simulink model "sampleModel4"  (R2022a)
settings: Solver=VariableStepAuto  StartTime=0.0  StopTime=10.0  RelTol=1e-3
undefined symbols (not defined in the file): DiscIntNeverNeededParam, magnitude, Newton, Raphson
libraries: simulink x90, slpidlib x34
(part 1 of 4)
settings Model: Creator=TSMC  LastModifiedBy=TSMC

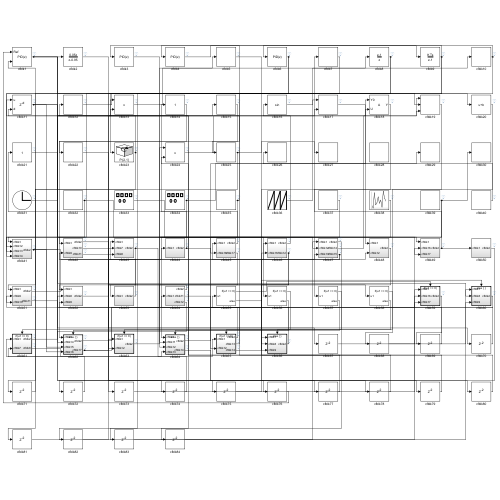
[thumbnail: Simulink's stored preview of the top-level diagram]
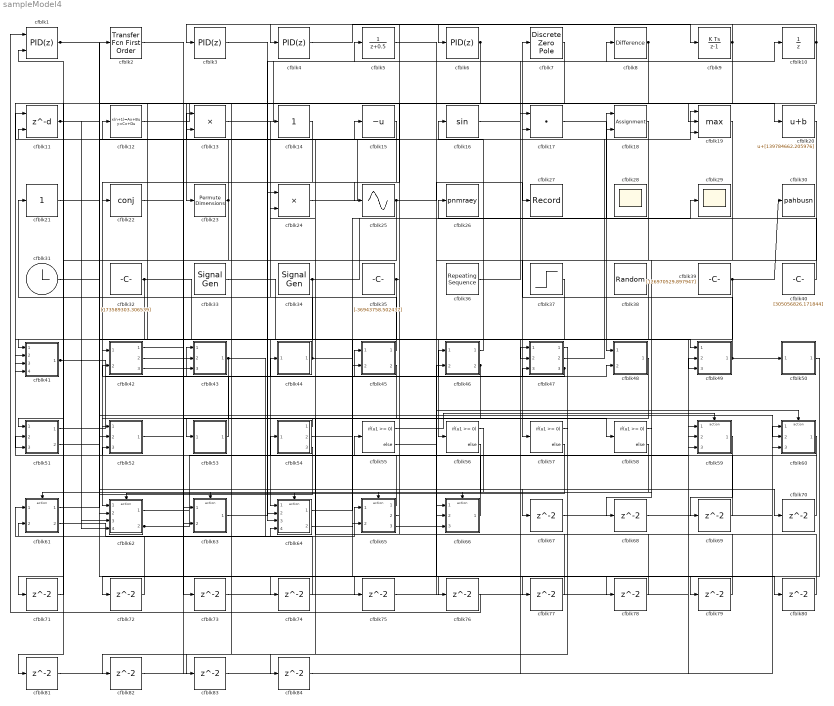
== system sampleModel4 ==
  cfblk1 : slpidlib/PID Controller (2DOF)  Controller=PID  Form=Parallel  TimeDomain=Discrete-time  UseExternalTs=off  SampleTime=1  IntegratorMethod=Forward Euler  FilterMethod=Forward Euler  ControllerParametersSource=internal  P=1  I=1  UseKiTs=off  D=0  N=100  UseFilter=on  b=1  c=1  TunerSelectOption=Transfer Function Based (PID Tuner App)  InitialConditionSource=internal  InitialConditionForIntegrator=0  InitialConditionForFilter=0  DifferentiatorICPrevScaledInput=0  ExternalReset=none  TrackingMode=off  Kt=1  LimitOutput=off  SatLimitsSource=internal  UpperSaturationLimit=inf  LowerSaturationLimit=-inf  LinearizeAsGain=off  AntiWindupMode=none  Kb=1  POutMin=[]  POutMax=[]  IOutMin=[]  IOutMax=[]  DOutMin=[]  DOutMax=[]  NOutMin=[]  NOutMax=[]  bOutMin=[]  bOutMax=[]  cOutMin=[]  cOutMax=[]  SumOutMin=[]  SumOutMax=[]  SaturationOutMin=[]  SaturationOutMax=[]  PParamMin=[]  PParamMax=[]  IParamMin=[]  IParamMax=[]  DParamMin=[]  DParamMax=[]  NParamMin=[]  NParamMax=[]  bParamMin=[]  bParamMax=[]  cParamMin=[]  cParamMax=[]  KbParamMin=[]  KbParamMax=[]  KtParamMin=[]  KtParamMax=[]  KbOutMin=[]  KbOutMax=[]  KtOutMin=[]  KtOutMax=[]  IntegratorOutMin=[]  IntegratorOutMax=[]  FilterOutMin=[]  FilterOutMax=[]  SumI1OutMin=[]  SumI1OutMax=[]  SumI2OutMin=[]  SumI2OutMax=[]  SumI3OutMin=[]  SumI3OutMax=[]  SumI4OutMin=[]  SumI4OutMax=[]  SumDOutMin=[]  SumDOutMax=[]  Sum1OutMin=[]  Sum1OutMax=[]  Sum2OutMin=[]  Sum2OutMax=[]  Sum3OutMin=[]  Sum3OutMax=[]  DifferentiatorOutMin=[]  DifferentiatorOutMax=[]  FilterDiffOutCoefMin=[]  FilterDiffOutCoefMax=[]  ReciprocalOutMin=[]  ReciprocalOutMax=[]  SumDenOutMin=[]  SumDenOutMax=[]  SumNumOutMin=[]  SumNumOutMax=[]  DivideOutMin=[]  DivideOutMax=[]  UdiffTsProdOutMin=[]  UdiffTsProdOutMax=[]  NTsProdOutMin=[]  NTsProdOutMax=[]  UintegralTsProdOutMin=[]  UintegralTsProdOutMax=[]  UngainTsProdOutMin=[]  UngainTsProdOutMax=[]  IntegratorContinuousStateAttributes=''  IntegratorStateMustResolveToSignalObject=off  IntegratorRTWStateStorageClass=Auto  FilterContinuousStateAttributes=''  FilterStateMustResolveToSignalObject=off  FilterRTWStateStorageClass=Auto  ParallelPVariant=InternalParameters  IdealPVariant=Disabled  IVariant=InternalParameters  DVariant=InternalParameters  bVariant=InternalParameters  cVariant=InternalParameters  IntegratorVariant=Discrete  SatVariant=Disabled  AWVariant=Passthrough  PCopyVariant=Disabled  TRVariant=Disabled  FdbkBlocksVariant=Forward  IdealPFdbkVariant=Disabled  SatFdbkVariant=Disabled  DerivativeFilterVariant=ForwardEulerFilter  NVariant=InternalParameters  NCopyVariant=Disabled  FilterICVariant=InternalICsFilter  IntegratorICVariant=InternalICs  ExternalResetVariant=Disabled  TRSumVariant=Passthrough  SumFdbkVariant=Disabled  SumVariant=Sum_PID  TsampFilterVariant=InternalTs  TsampNgainVariant=Passthrough  TsampIntegralVariant=Passthrough  ExternalSaturationOutDataTypeStr=Inherit: Same as second input
      settings: SourceProductBaseCode=SL
  cfblk10 : UnitDelay  HasFrameUpgradeWarning=on
  cfblk11 : Delay  DelayLengthSource=Input port  SampleTime=1
      settings: InputPortMap=u0,p1
  cfblk12 : DiscreteStateSpace
  cfblk13 : Product  Inputs=**
  cfblk14 : simulink/Math Operations/Slider Gain  gain=1  low=0  high=2
  cfblk15 : UnaryMinus
  cfblk16 : Trigonometry
  cfblk17 : DotProduct  OutDataTypeStr=Inherit: Inherit via internal rule
  cfblk18 : Assignment  DiagnosticForDimensions=Warning  IndexOptions=Index vector (dialog)  Indices=1  OutputSizes=1
  cfblk19 : MinMax  Function=max  Inputs=3
  cfblk2 : simulink/Discrete/Transfer Fcn First Order  PoleZ=0.95  ICPrevOutput=0.0  DoSatur=off
  cfblk20 : Bias  Bias=[139784662.205976]  SaturateOnIntegerOverflow=off
  cfblk21 : simulink/Math Operations/Slider Gain  gain=1  low=0  high=2
  cfblk22 : Math  Operator=conj
  cfblk23 : PermuteDimensions
  cfblk24 : Product  Inputs=**
  cfblk25 : Sin  TimeSource=Use external signal  SampleTime=0
  cfblk26 : ToWorkspace  VariableName=pnmraey  SaveFormat=Timeseries  SampleTime=-1
  cfblk27 : Record  FileSettingsInternal="{\"entries\":[{\"content\":{\"excelSettings\":{\"content\":{},\"type\":\"Streamout.ExcelSettings\"}},\"type\":\"Streamout.FileSettingStorage\",\"uuid\":\"17087479-7456-49d2-b213-c1ed72e334c6\"}],\"packageUris\":[\"http://schema.mathworks.com/mf0/streamout_blocks/R2020a\"],\"version\":\"1.0\"}"  SignalsInternal="{\"entries\":[{\"content\":{\"signals\":[{\"content\":{\"blockPath\":[\"sampleModel4/cfblk27\"],\"channel\":[],\"dimensions\":[1],\"domain\":\"sampleModel4/cfblk27\",\"lineColor\":\"#fe330a\",\"plots\":[1],\"port\":1,\"sid\":[\"\"],\"signalID\":1694,\"signalName\":\"cfblk25\"},\"type\":\"RecordBlkView.Signal\",\"uuid\":\"3c895155-84a9-4b62-997f-1b293a1a0065\"}]},\"type\":\"RecordBlkView.InputSignals\",\"uuid\":\"3ad74f41-9a96-40a9-a38d-74122b75e475\"}],\"packageUris\":[\"http://schema.mathworks.com/mf0/streamout_blocks/R2020a\"],\"version\":\"1.0\"}"  VisualizationBindings="{\"sparklinesplugin\":{\"info\":[{\"bindingParametersList\":[],\"subplotID\":1}]}}"
  cfblk28 : Scope
      settings: Floating=on
  cfblk29 : Scope
  cfblk3 : slpidlib/PID Controller  Controller=PID  Form=Parallel  TimeDomain=Discrete-time  UseExternalTs=off  SampleTime=1  IntegratorMethod=Forward Euler  FilterMethod=Forward Euler  ControllerParametersSource=internal  P=1  I=1  UseKiTs=off  D=0  N=100  UseFilter=on  TunerSelectOption=Transfer Function Based (PID Tuner App)  InitialConditionSource=internal  InitialConditionForIntegrator=0  InitialConditionForFilter=0  DifferentiatorICPrevScaledInput=0  ExternalReset=none  TrackingMode=off  Kt=1  LimitOutput=off  SatLimitsSource=internal  UpperSaturationLimit=inf  LowerSaturationLimit=-inf  LinearizeAsGain=off  AntiWindupMode=none  Kb=1  POutMin=[]  POutMax=[]  IOutMin=[]  IOutMax=[]  DOutMin=[]  DOutMax=[]  NOutMin=[]  NOutMax=[]  SumOutMin=[]  SumOutMax=[]  SaturationOutMin=[]  SaturationOutMax=[]  PParamMin=[]  PParamMax=[]  IParamMin=[]  IParamMax=[]  DParamMin=[]  DParamMax=[]  NParamMin=[]  NParamMax=[]  KbParamMin=[]  KbParamMax=[]  KtParamMin=[]  KtParamMax=[]  KbOutMin=[]  KbOutMax=[]  KtOutMin=[]  KtOutMax=[]  IntegratorOutMin=[]  IntegratorOutMax=[]  FilterOutMin=[]  FilterOutMax=[]  SumI1OutMin=[]  SumI1OutMax=[]  SumI2OutMin=[]  SumI2OutMax=[]  SumI3OutMin=[]  SumI3OutMax=[]  SumI4OutMin=[]  SumI4OutMax=[]  SumDOutMin=[]  SumDOutMax=[]  DifferentiatorOutMin=[]  DifferentiatorOutMax=[]  FilterDiffOutCoefMin=[]  FilterDiffOutCoefMax=[]  ReciprocalOutMin=[]  ReciprocalOutMax=[]  SumDenOutMin=[]  SumDenOutMax=[]  SumNumOutMin=[]  SumNumOutMax=[]  DivideOutMin=[]  DivideOutMax=[]  UdiffTsProdOutMin=[]  UdiffTsProdOutMax=[]  NTsProdOutMin=[]  NTsProdOutMax=[]  UintegralTsProdOutMin=[]  UintegralTsProdOutMax=[]  UngainTsProdOutMin=[]  UngainTsProdOutMax=[]  IntegratorContinuousStateAttributes=''  IntegratorStateMustResolveToSignalObject=off  IntegratorRTWStateStorageClass=Auto  FilterContinuousStateAttributes=''  FilterStateMustResolveToSignalObject=off  FilterRTWStateStorageClass=Auto  ParallelPVariant=InternalParameters  IdealPVariant=Disabled  IVariant=InternalParameters  DVariant=InternalParameters  IntegratorVariant=Discrete  SatVariant=Disabled  AWVariant=Passthrough  PCopyVariant=Disabled  TRVariant=Disabled  FdbkBlocksVariant=Forward  IdealPFdbkVariant=Disabled  SatFdbkVariant=Disabled  DerivativeFilterVariant=ForwardEulerFilter  NVariant=InternalParameters  NCopyVariant=Disabled  FilterICVariant=InternalICsFilter  IntegratorICVariant=InternalICs  ExternalResetVariant=Disabled  TRSumVariant=Passthrough  SumFdbkVariant=Disabled  SumVariant=Sum_PID  TsampFilterVariant=InternalTs  TsampNgainVariant=Passthrough  TsampIntegralVariant=Passthrough  ExternalSaturationOutDataTypeStr=Inherit: Same as second input  aMode=0
  cfblk30 : ToWorkspace  VariableName=pahbusn  SaveFormat=Timeseries  SampleTime=-1
  cfblk31 : Clock
  cfblk32 : Constant  Value=[173589303.306539]  SampleTime=1
  cfblk33 : SignalGenerator  WaveForm=square  Amplitude=[-172169984.241983]
  cfblk34 : SignalGenerator  WaveForm=square  Amplitude=[319821277.257385]
  cfblk35 : Constant  Value=[-36943758.502437]  SampleTime=1
  cfblk36 : simulink/Sources/Repeating Sequence  rep_seq_t=[0 2]  rep_seq_y=[462391417.037504, 938938528.441266]
  cfblk37 : Step  Time=[19.000000]  Before=[-522799793.188864]  After=[-514590504.970175]  SampleTime=0
  cfblk38 : UniformRandomNumber  Minimum=[-9810606010.362951]  Maximum=[9826531795.280075]  Seed=[80261952.000000]  SampleTime=0.1
  cfblk39 : Constant  Value=[126970529.897947]  SampleTime=1
  cfblk4 : slpidlib/PID Controller  Controller=PID  Form=Parallel  TimeDomain=Discrete-time  UseExternalTs=off  SampleTime=1  IntegratorMethod=Forward Euler  FilterMethod=Forward Euler  ControllerParametersSource=internal  P=1  I=1  UseKiTs=off  D=0  N=100  UseFilter=on  TunerSelectOption=Transfer Function Based (PID Tuner App)  InitialConditionSource=internal  InitialConditionForIntegrator=0  InitialConditionForFilter=0  DifferentiatorICPrevScaledInput=0  ExternalReset=none  TrackingMode=off  Kt=1  LimitOutput=off  SatLimitsSource=internal  UpperSaturationLimit=inf  LowerSaturationLimit=-inf  LinearizeAsGain=off  AntiWindupMode=none  Kb=1  POutMin=[]  POutMax=[]  IOutMin=[]  IOutMax=[]  DOutMin=[]  DOutMax=[]  NOutMin=[]  NOutMax=[]  SumOutMin=[]  SumOutMax=[]  SaturationOutMin=[]  SaturationOutMax=[]  PParamMin=[]  PParamMax=[]  IParamMin=[]  IParamMax=[]  DParamMin=[]  DParamMax=[]  NParamMin=[]  NParamMax=[]  KbParamMin=[]  KbParamMax=[]  KtParamMin=[]  KtParamMax=[]  KbOutMin=[]  KbOutMax=[]  KtOutMin=[]  KtOutMax=[]  IntegratorOutMin=[]  IntegratorOutMax=[]  FilterOutMin=[]  FilterOutMax=[]  SumI1OutMin=[]  SumI1OutMax=[]  SumI2OutMin=[]  SumI2OutMax=[]  SumI3OutMin=[]  SumI3OutMax=[]  SumI4OutMin=[]  SumI4OutMax=[]  SumDOutMin=[]  SumDOutMax=[]  DifferentiatorOutMin=[]  DifferentiatorOutMax=[]  FilterDiffOutCoefMin=[]  FilterDiffOutCoefMax=[]  ReciprocalOutMin=[]  ReciprocalOutMax=[]  SumDenOutMin=[]  SumDenOutMax=[]  SumNumOutMin=[]  SumNumOutMax=[]  DivideOutMin=[]  DivideOutMax=[]  UdiffTsProdOutMin=[]  UdiffTsProdOutMax=[]  NTsProdOutMin=[]  NTsProdOutMax=[]  UintegralTsProdOutMin=[]  UintegralTsProdOutMax=[]  UngainTsProdOutMin=[]  UngainTsProdOutMax=[]  IntegratorContinuousStateAttributes=''  IntegratorStateMustResolveToSignalObject=off  IntegratorRTWStateStorageClass=Auto  FilterContinuousStateAttributes=''  FilterStateMustResolveToSignalObject=off  FilterRTWStateStorageClass=Auto  ParallelPVariant=InternalParameters  IdealPVariant=Disabled  IVariant=InternalParameters  DVariant=InternalParameters  IntegratorVariant=Discrete  SatVariant=Disabled  AWVariant=Passthrough  PCopyVariant=Disabled  TRVariant=Disabled  FdbkBlocksVariant=Forward  IdealPFdbkVariant=Disabled  SatFdbkVariant=Disabled  DerivativeFilterVariant=ForwardEulerFilter  NVariant=InternalParameters  NCopyVariant=Disabled  FilterICVariant=InternalICsFilter  IntegratorICVariant=InternalICs  ExternalResetVariant=Disabled  TRSumVariant=Passthrough  SumFdbkVariant=Disabled  SumVariant=Sum_PID  TsampFilterVariant=InternalTs  TsampNgainVariant=Passthrough  TsampIntegralVariant=Passthrough  ExternalSaturationOutDataTypeStr=Inherit: Same as second input  aMode=0
  cfblk40 : Constant  Value=[305056826.171844]  SampleTime=1
  cfblk41 : Subsystem
  cfblk42 : Subsystem
  cfblk43 : Subsystem
  cfblk44 : Subsystem
  cfblk45 : Subsystem
  cfblk46 : Subsystem
  cfblk47 : Subsystem
  cfblk48 : Subsystem
  cfblk49 : Subsystem
  cfblk5 : DiscreteTransferFcn  SampleTime=1
  cfblk50 : Subsystem
  cfblk51 : Subsystem
  cfblk52 : Subsystem
  cfblk53 : Subsystem
  cfblk54 : Subsystem
  cfblk{55..58} (4 alike) : If  IfExpression=u1 >= 0  SampleTime=1
  cfblk59 : Subsystem  TreatAsAtomicUnit=on
  cfblk6 : slpidlib/PID Controller  Controller=PID  Form=Parallel  TimeDomain=Discrete-time  UseExternalTs=off  SampleTime=1  IntegratorMethod=Forward Euler  FilterMethod=Forward Euler  ControllerParametersSource=internal  P=1  I=1  UseKiTs=off  D=0  N=100  UseFilter=on  TunerSelectOption=Transfer Function Based (PID Tuner App)  InitialConditionSource=internal  InitialConditionForIntegrator=0  InitialConditionForFilter=0  DifferentiatorICPrevScaledInput=0  ExternalReset=none  TrackingMode=off  Kt=1  LimitOutput=off  SatLimitsSource=internal  UpperSaturationLimit=inf  LowerSaturationLimit=-inf  LinearizeAsGain=off  AntiWindupMode=none  Kb=1  POutMin=[]  POutMax=[]  IOutMin=[]  IOutMax=[]  DOutMin=[]  DOutMax=[]  NOutMin=[]  NOutMax=[]  SumOutMin=[]  SumOutMax=[]  SaturationOutMin=[]  SaturationOutMax=[]  PParamMin=[]  PParamMax=[]  IParamMin=[]  IParamMax=[]  DParamMin=[]  DParamMax=[]  NParamMin=[]  NParamMax=[]  KbParamMin=[]  KbParamMax=[]  KtParamMin=[]  KtParamMax=[]  KbOutMin=[]  KbOutMax=[]  KtOutMin=[]  KtOutMax=[]  IntegratorOutMin=[]  IntegratorOutMax=[]  FilterOutMin=[]  FilterOutMax=[]  SumI1OutMin=[]  SumI1OutMax=[]  SumI2OutMin=[]  SumI2OutMax=[]  SumI3OutMin=[]  SumI3OutMax=[]  SumI4OutMin=[]  SumI4OutMax=[]  SumDOutMin=[]  SumDOutMax=[]  DifferentiatorOutMin=[]  DifferentiatorOutMax=[]  FilterDiffOutCoefMin=[]  FilterDiffOutCoefMax=[]  ReciprocalOutMin=[]  ReciprocalOutMax=[]  SumDenOutMin=[]  SumDenOutMax=[]  SumNumOutMin=[]  SumNumOutMax=[]  DivideOutMin=[]  DivideOutMax=[]  UdiffTsProdOutMin=[]  UdiffTsProdOutMax=[]  NTsProdOutMin=[]  NTsProdOutMax=[]  UintegralTsProdOutMin=[]  UintegralTsProdOutMax=[]  UngainTsProdOutMin=[]  UngainTsProdOutMax=[]  IntegratorContinuousStateAttributes=''  IntegratorStateMustResolveToSignalObject=off  IntegratorRTWStateStorageClass=Auto  FilterContinuousStateAttributes=''  FilterStateMustResolveToSignalObject=off  FilterRTWStateStorageClass=Auto  ParallelPVariant=InternalParameters  IdealPVariant=Disabled  IVariant=InternalParameters  DVariant=InternalParameters  IntegratorVariant=Discrete  SatVariant=Disabled  AWVariant=Passthrough  PCopyVariant=Disabled  TRVariant=Disabled  FdbkBlocksVariant=Forward  IdealPFdbkVariant=Disabled  SatFdbkVariant=Disabled  DerivativeFilterVariant=ForwardEulerFilter  NVariant=InternalParameters  NCopyVariant=Disabled  FilterICVariant=InternalICsFilter  IntegratorICVariant=InternalICs  ExternalResetVariant=Disabled  TRSumVariant=Passthrough  SumFdbkVariant=Disabled  SumVariant=Sum_PID  TsampFilterVariant=InternalTs  TsampNgainVariant=Passthrough  TsampIntegralVariant=Passthrough  ExternalSaturationOutDataTypeStr=Inherit: Same as second input  aMode=0
  cfblk60 : Subsystem  TreatAsAtomicUnit=on
  cfblk61 : Subsystem  TreatAsAtomicUnit=on
  cfblk62 : Subsystem  TreatAsAtomicUnit=on
  cfblk63 : Subsystem  TreatAsAtomicUnit=on
  cfblk64 : Subsystem  TreatAsAtomicUnit=on
  cfblk65 : Subsystem  TreatAsAtomicUnit=on
  cfblk66 : Subsystem  TreatAsAtomicUnit=on
  cfblk{67..84} (18 alike) : Delay  SampleTime=1
  cfblk7 : DiscreteZeroPole  Poles=[0 0.5]  Gain=1
  cfblk8 : simulink/Discrete/Difference  ICPrevInput=0.0  OutMin=[]  OutMax=[]  OutDataTypeStr=Inherit: Inherit via back propagation  OutDataType=fixdt(1, 16)  OutScaling=2^-10  DoSatur=off
  cfblk9 : DiscreteIntegrator  ICPrevOutput=DiscIntNeverNeededParam  ICPrevScaledInput=DiscIntNeverNeededParam
  wires:
  cfblk34/1 -> cfblk64/1(cfblk1), cfblk18/1
  cfblk66/1(cfblk2) -> cfblk12/1
  cfblk43/1(cfblk2) -> cfblk65/1(cfblk1), cfblk63/2(cfblk12)
  cfblk13/1 -> cfblk5/1
  cfblk35/1 -> cfblk3/1, cfblk43/2(cfblk7)
  cfblk38/1 -> cfblk64/2(cfblk11)
  cfblk40/1 -> cfblk26/1
  cfblk45/1(cfblk2) -> cfblk14/1
  cfblk44/1(cfblk2) -> cfblk21/1, cfblk79/1
  cfblk8/1 -> cfblk23/1, cfblk81/1
  cfblk49/1(cfblk2) -> cfblk7/1, cfblk50/1(cfblk1)
  cfblk4/1 -> cfblk9/1
  cfblk14/1 -> cfblk62/1(cfblk1)
  cfblk32/1 -> cfblk56/1, cfblk41/4(cfblk14)
  cfblk18/1 -> cfblk57/1
  cfblk53/1(cfblk2) -> cfblk43/1(cfblk1)
  cfblk60/1(cfblk2) -> cfblk54/1(cfblk1)
  cfblk51/1(cfblk2) -> cfblk44/1(cfblk1)
  cfblk48/1(cfblk2) -> cfblk64/3(cfblk12)
  cfblk10/1 -> cfblk4/1, cfblk41/2(cfblk12)
  cfblk6/1 -> cfblk53/1(cfblk1), cfblk51/3(cfblk10)
  cfblk20/1 -> cfblk66/2(cfblk8)
  cfblk54/1(cfblk2) -> cfblk52/1(cfblk1)
  cfblk25/1 -> cfblk27/1, cfblk71/1
  cfblk52/1(cfblk2) -> cfblk46/1(cfblk1)
  cfblk17/1 -> cfblk48/1(cfblk1)
  cfblk36/1 -> cfblk17/1
  cfblk3/1 -> cfblk49/1(cfblk1)
  cfblk61/1(cfblk2) -> cfblk15/1
  cfblk54/2(cfblk11) -> cfblk65/2(cfblk12)
  cfblk24/1 -> cfblk19/1
  cfblk12/1 -> cfblk19/2
  cfblk47/2(cfblk14) -> cfblk19/3
  cfblk39/1 -> cfblk30/1, cfblk45/2(cfblk16), cfblk41/3(cfblk13)
  cfblk46/1(cfblk2) -> cfblk16/1
  cfblk2/1 -> cfblk58/1
  cfblk46/2(cfblk12) -> cfblk66/3(cfblk9), cfblk84/1
  cfblk61/2(cfblk8) -> cfblk64/4(cfblk13)
  cfblk31/1 -> cfblk2/1
  cfblk9/1 -> cfblk22/1, cfblk6/1, cfblk43/3(cfblk8)
  cfblk64/1(cfblk2) -> cfblk29/1
  cfblk37/1 -> cfblk41/1(cfblk1)
  cfblk62/1(cfblk2) -> cfblk49/2(cfblk16)
  cfblk63/1(cfblk2) -> cfblk8/1
  cfblk54/3(cfblk12) -> cfblk62/2(cfblk14)
  cfblk33/1 -> cfblk49/3(cfblk17)
  cfblk15/1 -> cfblk42/1(cfblk1)
  cfblk16/1 -> cfblk10/1
  cfblk1/1 -> cfblk60/2(cfblk8), cfblk20/1, cfblk47/2(cfblk12)
  cfblk23/1 -> cfblk13/1, cfblk51/1(cfblk1)
  cfblk62/2(cfblk17) -> cfblk24/1, cfblk18/2
  cfblk47/3(cfblk15) -> cfblk45/1(cfblk1), cfblk42/2(cfblk9)
  cfblk65/1(cfblk2) -> cfblk24/2
  cfblk65/2(cfblk13) -> cfblk11/2
  cfblk7/1 -> cfblk25/1
  cfblk65/3(cfblk14) -> cfblk48/2(cfblk12)
  cfblk41/1(cfblk2) -> cfblk13/2, cfblk62/3(cfblk15), cfblk47/3(cfblk13)
  cfblk11/1 -> cfblk62/4(cfblk16), cfblk17/2, cfblk70/1
  cfblk55/1 -> cfblk59/Action
  cfblk55/2 -> cfblk60/Action
  cfblk56/1 -> cfblk61/Action
  cfblk56/2 -> cfblk62/Action
  cfblk57/1 -> cfblk63/Action
  cfblk57/2 -> cfblk64/Action
  cfblk58/1 -> cfblk65/Action
  cfblk58/2 -> cfblk66/Action
  cfblk22/1 -> cfblk67/1
  cfblk67/1 -> cfblk60/1(cfblk1)
  cfblk19/1 -> cfblk68/1
  cfblk68/1 -> cfblk59/1(cfblk1)
  cfblk59/1(cfblk2) -> cfblk69/1
  cfblk69/1 -> cfblk52/2(cfblk8)
  cfblk70/1 -> cfblk52/3(cfblk9)
  cfblk71/1 -> cfblk1/2
  cfblk50/1(cfblk2) -> cfblk72/1
  cfblk72/1 -> cfblk61/1(cfblk1)
  cfblk42/1(cfblk2) -> cfblk73/1
  cfblk73/1 -> cfblk59/3(cfblk17)
  cfblk42/2(cfblk10) -> cfblk74/1
  cfblk74/1 -> cfblk61/2(cfblk7)
  cfblk42/3(cfblk11) -> cfblk75/1
  cfblk75/1 -> cfblk46/2(cfblk11)
  cfblk64/2(cfblk14) -> cfblk76/1
  cfblk76/1 -> cfblk1/1
  cfblk5/1 -> cfblk77/1
  cfblk77/1 -> cfblk11/1
  cfblk21/1 -> cfblk78/1
  cfblk78/1 -> cfblk55/1
  cfblk79/1 -> cfblk51/2(cfblk9)
  cfblk51/2(cfblk11) -> cfblk80/1
  cfblk80/1 -> cfblk66/1(cfblk1)
  cfblk81/1 -> cfblk63/1(cfblk1)
  cfblk47/1(cfblk2) -> cfblk82/1
  cfblk82/1 -> cfblk59/2(cfblk16)
  cfblk45/2(cfblk17) -> cfblk83/1
  cfblk83/1 -> cfblk47/1(cfblk1)
  cfblk84/1 -> cfblk60/3(cfblk9)

== system sampleModel4/cfblk41 ==
  cfblk1 : Inport
  cfblk12 : Inport  Port=2
  cfblk13 : Inport  Port=3
  cfblk14 : Inport  Port=4
  cfblk10 : Subsystem
  cfblk11 : Subsystem
  cfblk15 : Delay  SampleTime=1
  cfblk3 : Delay  DelayLengthSource=Input port  SampleTime=1
      settings: InputPortMap=u0,p1
  cfblk4 : simulink/Discrete/Tapped Delay  vinit=0.0  samptime=-1  NumDelays=1  DelayOrder=Oldest  includeCurrent=off
  cfblk5 : DiscreteFilter  SampleTime=1
  cfblk6 : Squeeze
  cfblk7 : Squeeze
  cfblk8 : Sum  Inputs=+
  cfblk9 : Constant  Value=[257371044.313434]  SampleTime=1
  cfblk2 : Outport
  wires:
  cfblk11/1(cfblk2) -> cfblk8/1
  cfblk10/1(cfblk2) -> cfblk7/1
  cfblk7/1 -> cfblk11/1(cfblk1)
  cfblk14/1 -> cfblk4/1
  cfblk4/1 -> cfblk2/1
  cfblk12/1 -> cfblk3/1
  cfblk8/1 -> cfblk3/2
  cfblk5/1 -> cfblk10/1(cfblk1)
  cfblk13/1 -> cfblk10/2(cfblk16)
  cfblk10/2(cfblk17) -> cfblk11/2(cfblk10)
  cfblk1/1 -> cfblk6/1
  cfblk11/2(cfblk11) -> cfblk15/1
  cfblk15/1 -> cfblk5/1

== system sampleModel4/cfblk42 ==
  cfblk1 : Inport
  cfblk9 : Inport  Port=2
  cfblk12 : Delay  SampleTime=1
  cfblk3 : simulink/Discrete/Transfer Fcn Real Zero  ZeroZ=0.75  ICPrevInput=0.0  DoSatur=off
      settings: SourceProductBaseCode=SL
  cfblk4 : Sum  Inputs=+-
  cfblk5 : Product  Inputs=*
  cfblk6 : Constant  Value=[-85523003.532124]  SampleTime=1
  cfblk7 : Subsystem
  cfblk8 : Subsystem
  cfblk2 : Outport
  cfblk10 : Outport  Port=2
  cfblk11 : Outport  Port=3
  wires:
  cfblk8/1(cfblk2) -> cfblk7/1(cfblk1)
  cfblk4/1 -> cfblk8/1(cfblk1)
  cfblk1/1 -> cfblk3/1
  cfblk9/1 -> cfblk2/1
  cfblk6/1 -> cfblk8/2(cfblk11)
  cfblk3/1 -> cfblk4/1
  cfblk5/1 -> cfblk10/1, cfblk12/1
  cfblk7/1(cfblk2) -> cfblk5/1
  cfblk8/2(cfblk12) -> cfblk7/2(cfblk9)
  cfblk8/3(cfblk13) -> cfblk7/3(cfblk10)
  cfblk8/4(cfblk14) -> cfblk11/1
  cfblk12/1 -> cfblk4/2

== system sampleModel4/cfblk43 ==
  cfblk1 : Inport
  cfblk7 : Inport  Port=2
  cfblk8 : Inport  Port=3
  cfblk3 : DotProduct  OutDataTypeStr=Inherit: Inherit via internal rule
  cfblk4 : Sum  Inputs=+-
  cfblk5 : Polyval  Coefs=[ +2.081618890e-019, -1.441693666e-014, +4.719686976e-010, -8.536869453e-006, +1.621573104e-001, -8.087801117e+001 ]
  cfblk6 : Constant  Value=[971477351.565452]  SampleTime=1
  cfblk9 : Delay  SampleTime=1
  cfblk2 : Outport
  wires:
  cfblk4/1 -> cfblk5/1
  cfblk5/1 -> cfblk3/1
  cfblk8/1 -> cfblk2/1
  cfblk7/1 -> cfblk3/2
  cfblk1/1 -> cfblk4/2
  cfblk3/1 -> cfblk9/1
  cfblk9/1 -> cfblk4/1

== system sampleModel4/cfblk44 ==
  cfblk1 : Inport
  cfblk10 : Delay  SampleTime=1
  cfblk3 : Sqrt
  cfblk4 : Gain  Gain=[-78770350.999530]
  cfblk5 : Subsystem
  cfblk6 : Subsystem
  cfblk7 : Subsystem
  cfblk8 : Delay  SampleTime=1
  cfblk9 : Delay  SampleTime=1
  cfblk2 : Outport
  wires:
  cfblk7/1(cfblk2) -> cfblk5/3(cfblk11), cfblk5/4(cfblk12), cfblk5/5(cfblk13), cfblk8/1
  cfblk5/1(cfblk2) -> cfblk4/1
  cfblk1/1 -> cfblk6/2(cfblk14), cfblk3/1, cfblk5/2(cfblk10), cfblk5/6(cfblk14)
  cfblk6/1(cfblk2) -> cfblk7/1(cfblk1)
  cfblk3/1 -> cfblk5/1(cfblk1), cfblk5/7(cfblk15)
  cfblk4/1 -> cfblk2/1
  cfblk6/2(cfblk17) -> cfblk7/2(cfblk7)
  cfblk8/1 -> cfblk6/1(cfblk1)
  cfblk5/2(cfblk16) -> cfblk9/1
  cfblk9/1 -> cfblk6/3(cfblk15)
  cfblk5/3(cfblk17) -> cfblk10/1
  cfblk10/1 -> cfblk6/4(cfblk16)

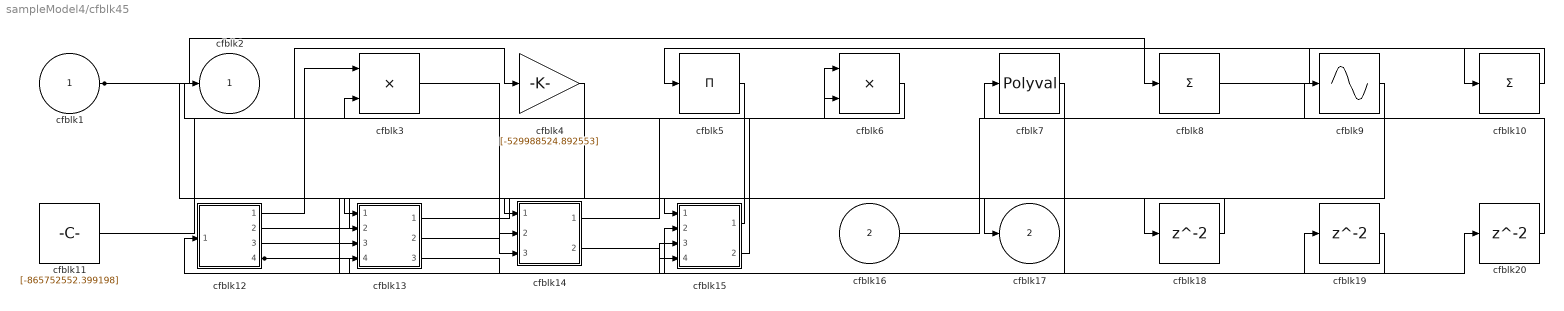
== system sampleModel4/cfblk45 ==
  cfblk1 : Inport
  cfblk16 : Inport  Port=2
  cfblk10 : Sum  Inputs=+
  cfblk11 : Constant  Value=[-865752552.399198]  SampleTime=1
  cfblk12 : Subsystem
  cfblk13 : Subsystem
  cfblk14 : Subsystem
  cfblk15 : Subsystem
  cfblk18 : Delay  SampleTime=1
  cfblk19 : Delay  SampleTime=1
  cfblk20 : Delay  SampleTime=1
  cfblk3 : Product  Inputs=**
  cfblk4 : Gain  Gain=[-529988524.892553]
  cfblk5 : Product  Inputs=*
  cfblk6 : Product
  cfblk7 : Polyval  Coefs=[ +2.081618890e-019, -1.441693666e-014, +4.719686976e-010, -8.536869453e-006, +1.621573104e-001, -8.087801117e+001 ]
  cfblk8 : Sum  Inputs=+
  cfblk9 : Sin  TimeSource=Use external signal  SampleTime=0
  cfblk2 : Outport
  cfblk17 : Outport  Port=2
  wires:
  cfblk12/1(cfblk2) -> cfblk3/1
  cfblk11/1 -> cfblk4/1
  cfblk7/1 -> cfblk12/1(cfblk1)
  cfblk8/1 -> cfblk10/1
  cfblk12/2(cfblk9) -> cfblk15/1(cfblk1)
  cfblk15/1(cfblk2) -> cfblk13/1(cfblk1)
  cfblk13/1(cfblk2) -> cfblk17/1
  cfblk1/1 -> cfblk8/1, cfblk13/3(cfblk14)
  cfblk15/2(cfblk14) -> cfblk2/1
  cfblk12/4(cfblk11) -> cfblk15/2(cfblk11), cfblk13/4(cfblk15)
  cfblk16/1 -> cfblk9/1
  cfblk6/1 -> cfblk3/2
  cfblk10/1 -> cfblk5/1
  cfblk5/1 -> cfblk14/2(cfblk8)
  cfblk14/1(cfblk2) -> cfblk6/1
  cfblk13/2(cfblk16) -> cfblk6/2
  cfblk9/1 -> cfblk13/2(cfblk13)
  cfblk4/1 -> cfblk14/3(cfblk9)
  cfblk14/2(cfblk10) -> cfblk15/4(cfblk13)
  cfblk3/1 -> cfblk18/1
  cfblk18/1 -> cfblk14/1(cfblk1)
  cfblk13/3(cfblk17) -> cfblk19/1
  cfblk19/1 -> cfblk15/3(cfblk12)
  cfblk12/3(cfblk10) -> cfblk20/1
  cfblk20/1 -> cfblk7/1

== system sampleModel4/cfblk46 ==
  cfblk1 : Inport
  cfblk11 : Inport  Port=2
  cfblk10 : Subsystem
  cfblk13 : Delay  SampleTime=1
  cfblk3 : Delay  DelayLengthSource=Input port  SampleTime=1
      settings: InputPortMap=u0,p1
  cfblk4 : slpidlib/PID Controller (2DOF)  Controller=PID  Form=Parallel  TimeDomain=Discrete-time  UseExternalTs=off  SampleTime=1  IntegratorMethod=Forward Euler  FilterMethod=Forward Euler  ControllerParametersSource=internal  P=1  I=1  UseKiTs=off  D=0  N=100  UseFilter=on  b=1  c=1  TunerSelectOption=Transfer Function Based (PID Tuner App)  InitialConditionSource=internal  InitialConditionForIntegrator=0  InitialConditionForFilter=0  DifferentiatorICPrevScaledInput=0  ExternalReset=none  TrackingMode=off  Kt=1  LimitOutput=off  SatLimitsSource=internal  UpperSaturationLimit=inf  LowerSaturationLimit=-inf  LinearizeAsGain=off  AntiWindupMode=none  Kb=1  POutMin=[]  POutMax=[]  IOutMin=[]  IOutMax=[]  DOutMin=[]  DOutMax=[]  NOutMin=[]  NOutMax=[]  bOutMin=[]  bOutMax=[]  cOutMin=[]  cOutMax=[]  SumOutMin=[]  SumOutMax=[]  SaturationOutMin=[]  SaturationOutMax=[]  PParamMin=[]  PParamMax=[]  IParamMin=[]  IParamMax=[]  DParamMin=[]  DParamMax=[]  NParamMin=[]  NParamMax=[]  bParamMin=[]  bParamMax=[]  cParamMin=[]  cParamMax=[]  KbParamMin=[]  KbParamMax=[]  KtParamMin=[]  KtParamMax=[]  KbOutMin=[]  KbOutMax=[]  KtOutMin=[]  KtOutMax=[]  IntegratorOutMin=[]  IntegratorOutMax=[]  FilterOutMin=[]  FilterOutMax=[]  SumI1OutMin=[]  SumI1OutMax=[]  SumI2OutMin=[]  SumI2OutMax=[]  SumI3OutMin=[]  SumI3OutMax=[]  SumI4OutMin=[]  SumI4OutMax=[]  SumDOutMin=[]  SumDOutMax=[]  Sum1OutMin=[]  Sum1OutMax=[]  Sum2OutMin=[]  Sum2OutMax=[]  Sum3OutMin=[]  Sum3OutMax=[]  DifferentiatorOutMin=[]  DifferentiatorOutMax=[]  FilterDiffOutCoefMin=[]  FilterDiffOutCoefMax=[]  ReciprocalOutMin=[]  ReciprocalOutMax=[]  SumDenOutMin=[]  SumDenOutMax=[]  SumNumOutMin=[]  SumNumOutMax=[]  DivideOutMin=[]  DivideOutMax=[]  UdiffTsProdOutMin=[]  UdiffTsProdOutMax=[]  NTsProdOutMin=[]  NTsProdOutMax=[]  UintegralTsProdOutMin=[]  UintegralTsProdOutMax=[]  UngainTsProdOutMin=[]  UngainTsProdOutMax=[]  IntegratorContinuousStateAttributes=''  IntegratorStateMustResolveToSignalObject=off  IntegratorRTWStateStorageClass=Auto  FilterContinuousStateAttributes=''  FilterStateMustResolveToSignalObject=off  FilterRTWStateStorageClass=Auto  ParallelPVariant=InternalParameters  IdealPVariant=Disabled  IVariant=InternalParameters  DVariant=InternalParameters  bVariant=InternalParameters  cVariant=InternalParameters  IntegratorVariant=Discrete  SatVariant=Disabled  AWVariant=Passthrough  PCopyVariant=Disabled  TRVariant=Disabled  FdbkBlocksVariant=Forward  IdealPFdbkVariant=Disabled  SatFdbkVariant=Disabled  DerivativeFilterVariant=ForwardEulerFilter  NVariant=InternalParameters  NCopyVariant=Disabled  FilterICVariant=InternalICsFilter  IntegratorICVariant=InternalICs  ExternalResetVariant=Disabled  TRSumVariant=Passthrough  SumFdbkVariant=Disabled  SumVariant=Sum_PID  TsampFilterVariant=InternalTs  TsampNgainVariant=Passthrough  TsampIntegralVariant=Passthrough  ExternalSaturationOutDataTypeStr=Inherit: Same as second input
      settings: SourceProductBaseCode=SL
  cfblk5 : simulink/Discrete/Transfer Fcn First Order  PoleZ=0.95  ICPrevOutput=0.0  DoSatur=off
  cfblk6 : simulink/Math Operations/Slider Gain  gain=1  low=0  high=2
  cfblk7 : Constant  Value=[951840186.226088]  SampleTime=1
  cfblk8 : Constant  Value=[-297993001.086612]  SampleTime=1
  cfblk9 : Subsystem
  cfblk2 : Outport
  cfblk12 : Outport  Port=2
  wires:
  cfblk3/1 -> cfblk2/1, cfblk10/3(cfblk11), cfblk13/1
  cfblk9/1(cfblk2) -> cfblk10/1(cfblk1), cfblk4/2
  cfblk4/1 -> cfblk5/1
  cfblk1/1 -> cfblk9/1(cfblk1)
  cfblk11/1 -> cfblk3/1, cfblk10/4(cfblk12)
  cfblk10/1(cfblk2) -> cfblk6/1
  cfblk7/1 -> cfblk4/1
  cfblk6/1 -> cfblk12/1
  cfblk8/1 -> cfblk10/2(cfblk10)
  cfblk5/1 -> cfblk3/2
  cfblk13/1 -> cfblk9/2(cfblk8)

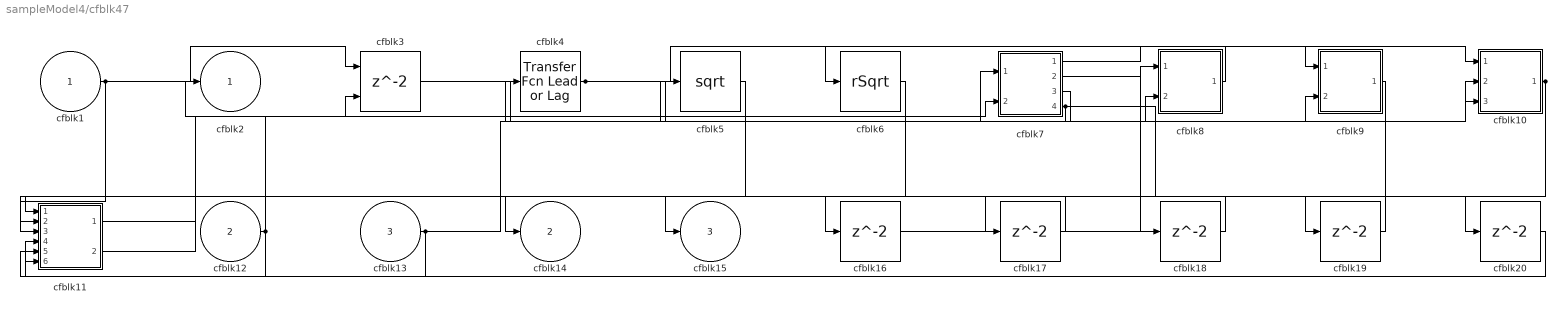
== system sampleModel4/cfblk47 ==
  cfblk1 : Inport
  cfblk12 : Inport  Port=2
  cfblk13 : Inport  Port=3
  cfblk10 : Subsystem
  cfblk11 : Subsystem
  cfblk{16..20} (5 alike) : Delay  SampleTime=1
  cfblk3 : Delay  ShowEnablePort=on  SampleTime=1
      settings: InputPortMap=u0,e6
  cfblk4 : simulink/Discrete/Transfer Fcn Lead or Lag  PoleZ=0.95  ZeroZ=0.75  ICPrevOutput=0.0  ICPrevInput=0.0  DoSatur=off
      settings: SourceProductBaseCode=SL
  cfblk5 : Sqrt
  cfblk6 : Sqrt  Operator=rSqrt  AlgorithmType=Newton-Raphson
  cfblk7 : Subsystem
  cfblk8 : Subsystem
  cfblk9 : Subsystem
  cfblk2 : Outport
  cfblk14 : Outport  Port=2
  cfblk15 : Outport  Port=3
  wires:
  cfblk4/1 -> cfblk9/1(cfblk1), cfblk10/3(cfblk9)
  cfblk1/1 -> cfblk3/1, cfblk11/3(cfblk13)
  cfblk10/1(cfblk2) -> cfblk15/1, cfblk17/1
  cfblk12/1 -> cfblk2/1, cfblk11/4(cfblk14)
  cfblk3/1 -> cfblk8/2(cfblk7)
  cfblk5/1 -> cfblk14/1
  cfblk13/1 -> cfblk9/2(cfblk10), cfblk10/2(cfblk8), cfblk11/6(cfblk16)
  cfblk8/1(cfblk2) -> cfblk6/1
  cfblk11/1(cfblk2) -> cfblk7/2(cfblk10)
  cfblk7/1(cfblk2) -> cfblk10/1(cfblk1)
  cfblk11/2(cfblk17) -> cfblk3/2
  cfblk7/3(cfblk12) -> cfblk4/1
  cfblk7/4(cfblk13) -> cfblk5/1, cfblk20/1
  cfblk6/1 -> cfblk16/1
  cfblk16/1 -> cfblk8/1(cfblk1)
  cfblk17/1 -> cfblk11/2(cfblk12)
  cfblk7/2(cfblk11) -> cfblk18/1
  cfblk18/1 -> cfblk11/1(cfblk1)
  cfblk9/1(cfblk2) -> cfblk19/1
  cfblk19/1 -> cfblk7/1(cfblk1)
  cfblk20/1 -> cfblk11/5(cfblk15)

== system sampleModel4/cfblk48 ==
  cfblk1 : Inport
  cfblk12 : Inport  Port=2
  cfblk10 : Subsystem
  cfblk11 : Subsystem
  cfblk{13..16} (4 alike) : Delay  SampleTime=1
  cfblk3 : simulink/Discrete/Transfer Fcn Real Zero  ZeroZ=0.75  ICPrevInput=0.0  DoSatur=off
      settings: SourceProductBaseCode=SL
  cfblk4 : simulink/Discrete/Transfer Fcn First Order  PoleZ=0.95  ICPrevOutput=0.0  DoSatur=off
  cfblk5 : Sqrt
  cfblk6 : simulink/Math Operations/MinMax Running Resettable  Function=min  vinit=0.0
  cfblk7 : ComplexToMagnitudeAngle
  cfblk8 : Subsystem
  cfblk9 : Subsystem
  cfblk2 : Outport
  wires:
  cfblk1/1 -> cfblk4/1
  cfblk3/1 -> cfblk6/1
  cfblk5/1 -> cfblk11/3(cfblk8), cfblk13/1
  cfblk4/1 -> cfblk10/2(cfblk11)
  cfblk6/1 -> cfblk5/1
  cfblk11/1(cfblk2) -> cfblk8/2(cfblk8), cfblk14/1
  cfblk12/1 -> cfblk11/1(cfblk1), cfblk8/1(cfblk1), cfblk8/3(cfblk9)
  cfblk7/1 -> cfblk9/1(cfblk1)
  cfblk10/1(cfblk2) -> cfblk2/1
  cfblk8/1(cfblk2) -> cfblk7/1
  cfblk10/2(cfblk14) -> cfblk6/2
  cfblk10/3(cfblk15) -> cfblk3/1
  cfblk13/1 -> cfblk10/1(cfblk1)
  cfblk14/1 -> cfblk10/3(cfblk12)
  cfblk9/1(cfblk2) -> cfblk15/1
  cfblk15/1 -> cfblk10/4(cfblk13)
  cfblk7/2 -> cfblk16/1
  cfblk16/1 -> cfblk11/2(cfblk7)

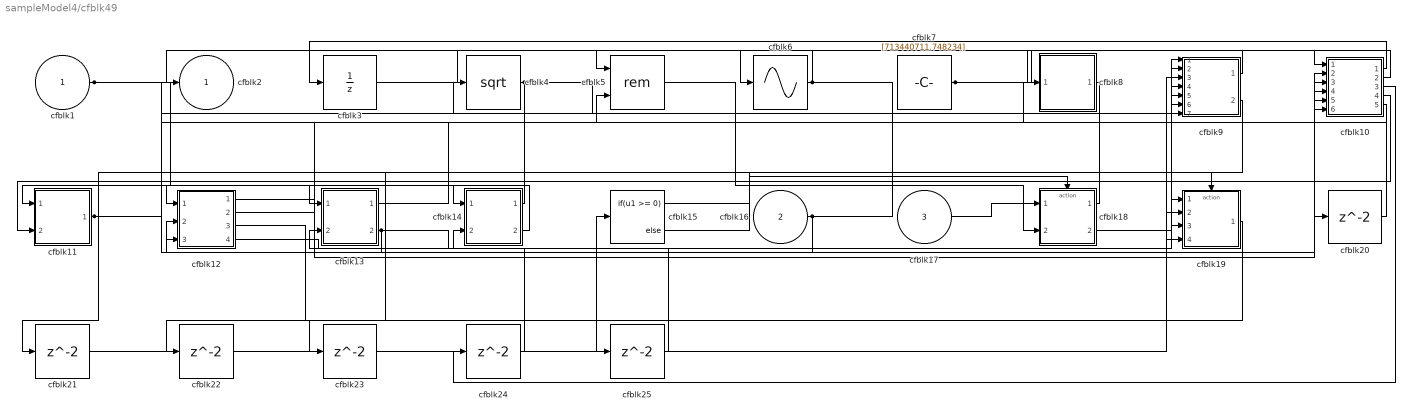
== system sampleModel4/cfblk49 ==
  cfblk1 : Inport
  cfblk16 : Inport  Port=2
  cfblk17 : Inport  Port=3
  cfblk10 : Subsystem
  cfblk11 : Subsystem
  cfblk12 : Subsystem
  cfblk13 : Subsystem
  cfblk14 : Subsystem
  cfblk15 : If  IfExpression=u1 >= 0  SampleTime=1
  cfblk18 : Subsystem  TreatAsAtomicUnit=on
  cfblk19 : Subsystem  TreatAsAtomicUnit=on
  cfblk{20..25} (6 alike) : Delay  SampleTime=1
  cfblk3 : UnitDelay  HasFrameUpgradeWarning=on
  cfblk4 : Sqrt
  cfblk5 : Math  Operator=rem
  cfblk6 : Sin  TimeSource=Use external signal  SampleTime=0
  cfblk7 : Constant  Value=[713440711.748234]  SampleTime=1
  cfblk8 : Subsystem
  cfblk9 : Subsystem
  cfblk2 : Outport
  wires:
  cfblk7/1 -> cfblk10/1(cfblk1), cfblk10/6(cfblk13)
  cfblk3/1 -> cfblk5/1
  cfblk18/1(cfblk2) -> cfblk4/1
  cfblk1/1 -> cfblk14/1(cfblk1), cfblk10/5(cfblk12)
  cfblk17/1 -> cfblk18/1(cfblk1)
  cfblk9/1(cfblk2) -> cfblk8/1(cfblk1)
  cfblk10/1(cfblk2) -> cfblk3/1
  cfblk18/2(cfblk14) -> cfblk9/1(cfblk1)
  cfblk16/1 -> cfblk9/2(cfblk10), cfblk12/2(cfblk11)
  cfblk10/2(cfblk14) -> cfblk6/1
  cfblk12/1(cfblk2) -> cfblk10/2(cfblk9)
  cfblk4/1 -> cfblk11/1(cfblk1), cfblk9/5(cfblk13)
  cfblk12/2(cfblk13) -> cfblk10/3(cfblk10)
  cfblk6/1 -> cfblk2/1, cfblk9/6(cfblk14), cfblk9/7(cfblk15)
  cfblk5/1 -> cfblk18/2(cfblk13)
  cfblk11/1(cfblk2) -> cfblk9/4(cfblk12), cfblk20/1
  cfblk13/1(cfblk2) -> cfblk10/4(cfblk11)
  cfblk14/1(cfblk2) -> cfblk13/1(cfblk1)
  cfblk12/4(cfblk15) -> cfblk19/1(cfblk1)
  cfblk14/2(cfblk15) -> cfblk12/1(cfblk1)
  cfblk10/4(cfblk16) -> cfblk11/2(cfblk10)
  cfblk13/2(cfblk9) -> cfblk19/3(cfblk10), cfblk12/3(cfblk12)
  cfblk10/5(cfblk17) -> cfblk19/4(cfblk11)
  cfblk15/1 -> cfblk18/Action
  cfblk15/2 -> cfblk19/Action
  cfblk20/1 -> cfblk5/2
  cfblk8/1(cfblk2) -> cfblk21/1
  cfblk21/1 -> cfblk15/1
  cfblk19/1(cfblk2) -> cfblk22/1
  cfblk22/1 -> cfblk9/3(cfblk11)
  cfblk9/2(cfblk16) -> cfblk23/1
  cfblk23/1 -> cfblk19/2(cfblk9)
  cfblk10/3(cfblk15) -> cfblk24/1
  cfblk24/1 -> cfblk13/2(cfblk8)
  cfblk12/3(cfblk14) -> cfblk25/1
  cfblk25/1 -> cfblk14/2(cfblk14)

== system sampleModel4/cfblk50 ==
  cfblk1 : Inport
  cfblk10 : Subsystem
  cfblk11 : Delay  SampleTime=1
  cfblk12 : Delay  SampleTime=1
  cfblk13 : Delay  SampleTime=1
  cfblk3 : simulink/Discrete/Transfer Fcn Lead or Lag  PoleZ=0.95  ZeroZ=0.75  ICPrevOutput=0.0  ICPrevInput=0.0  DoSatur=off
      settings: SourceProductBaseCode=SL
  cfblk4 : simulink/Discrete/Transfer Fcn First Order  PoleZ=0.95  ICPrevOutput=0.0  DoSatur=off
  cfblk5 : Product  Inputs=**
  cfblk6 : simulink/Math Operations/MinMax Running Resettable  Function=min  vinit=0.0
  cfblk7 : Sin  TimeSource=Use external signal  SampleTime=0
  cfblk8 : Assignment  DiagnosticForDimensions=Warning  IndexOptions=Index vector (dialog)  Indices=1  OutputSizes=1
  cfblk9 : Subsystem
  cfblk2 : Outport
  wires:
  cfblk4/1 -> cfblk3/1, cfblk10/1(cfblk1)
  cfblk1/1 -> cfblk8/2
  cfblk9/2(cfblk14) -> cfblk6/1, cfblk6/2
  cfblk6/1 -> cfblk4/1, cfblk10/3(cfblk7)
  cfblk7/1 -> cfblk2/1
  cfblk3/1 -> cfblk7/1, cfblk12/1
  cfblk5/1 -> cfblk9/2(cfblk11)
  cfblk8/1 -> cfblk9/3(cfblk12), cfblk5/1, cfblk10/2(cfblk6), cfblk5/2
  cfblk9/1(cfblk2) -> cfblk11/1
  cfblk11/1 -> cfblk8/1
  cfblk12/1 -> cfblk9/4(cfblk13)
  cfblk10/1(cfblk2) -> cfblk13/1
  cfblk13/1 -> cfblk9/1(cfblk1)

== system sampleModel4/cfblk51 ==
  cfblk1 : Inport
  cfblk9 : Inport  Port=2
  cfblk10 : Inport  Port=3
  cfblk12 : Delay  SampleTime=1
  cfblk13 : Delay  SampleTime=1
  cfblk3 : Squeeze
  cfblk4 : Sum  Inputs=+-
  cfblk5 : Bias  Bias=[-298897600.256370]  SaturateOnIntegerOverflow=off
  cfblk6 : Constant  Value=[811273915.710360]  SampleTime=1
  cfblk7 : Subsystem
  cfblk8 : Subsystem
  cfblk2 : Outport
  cfblk11 : Outport  Port=2
  wires:
  cfblk6/1 -> cfblk7/1(cfblk1)
  cfblk3/1 -> cfblk4/1
  cfblk9/1 -> cfblk2/1
  cfblk4/1 -> cfblk5/1
  cfblk7/1(cfblk2) -> cfblk12/1, cfblk13/1
  cfblk1/1 -> cfblk3/1, cfblk4/2
  cfblk10/1 -> cfblk8/2(cfblk11)
  cfblk5/1 -> cfblk8/3(cfblk12)
  cfblk8/1(cfblk2) -> cfblk11/1, cfblk7/2(cfblk7)
  cfblk12/1 -> cfblk8/1(cfblk1)
  cfblk13/1 -> cfblk8/4(cfblk13)

== system sampleModel4/cfblk52 ==
  cfblk1 : Inport
  cfblk8 : Inport  Port=2
  cfblk9 : Inport  Port=3
  cfblk10 : Delay  SampleTime=1
  cfblk3 : DiscreteFilter  SampleTime=1
  cfblk4 : DiscreteFilter  SampleTime=1
  cfblk5 : Polyval  Coefs=[ +2.081618890e-019, -1.441693666e-014, +4.719686976e-010, -8.536869453e-006, +1.621573104e-001, -8.087801117e+001 ]
  cfblk6 : MinMax  Function=max  Inputs=2
  cfblk7 : Subsystem
  cfblk2 : Outport
  wires:
  cfblk1/1 -> cfblk3/1
  cfblk3/1 -> cfblk5/1, cfblk7/2(cfblk9), cfblk7/3(cfblk10), cfblk7/4(cfblk11), cfblk7/5(cfblk12)
  cfblk9/1 -> cfblk6/1
  cfblk4/1 -> cfblk6/2
  cfblk8/1 -> cfblk2/1
  cfblk5/1 -> cfblk7/1(cfblk1)
  cfblk6/1 -> cfblk10/1
  cfblk10/1 -> cfblk4/1

== system sampleModel4/cfblk53 ==
  cfblk1 : Inport
  cfblk{8..13} (6 alike) : Delay  SampleTime=1
  cfblk3 : PermuteDimensions
  cfblk4 : Product
  cfblk5 : Gain  Gain=[366053708.136588]
  cfblk6 : Subsystem
  cfblk7 : Subsystem
  cfblk2 : Outport
  wires:
  cfblk5/1 -> cfblk3/1
  cfblk4/1 -> cfblk7/1(cfblk1), cfblk13/1
  cfblk3/1 -> cfblk8/1, cfblk9/1, cfblk10/1
  cfblk6/1(cfblk2) -> cfblk4/2
  cfblk6/2(cfblk17) -> cfblk7/2(cfblk11), cfblk2/1
  cfblk7/1(cfblk2) -> cfblk5/1, cfblk11/1, cfblk12/1
  cfblk1/1 -> cfblk6/1(cfblk1)
  cfblk8/1 -> cfblk4/1
  cfblk9/1 -> cfblk7/3(cfblk12)
  cfblk10/1 -> cfblk7/4(cfblk13)
  cfblk11/1 -> cfblk6/2(cfblk14)
  cfblk12/1 -> cfblk6/3(cfblk15)
  cfblk13/1 -> cfblk6/4(cfblk16)

== system sampleModel4/cfblk54 ==
  cfblk1 : Inport
  cfblk10 : Subsystem
  cfblk{13..16} (4 alike) : Delay  SampleTime=1
  cfblk3 : DiscreteStateSpace
  cfblk4 : Math  Operator=10^u
  cfblk5 : simulink/Math Operations/MinMax Running Resettable  Function=min  vinit=0.0
  cfblk6 : Constant  Value=[89699818.959386]  SampleTime=1
  cfblk7 : Constant  Value=[-625989660.662370]  SampleTime=1
  cfblk8 : Subsystem
  cfblk9 : Subsystem
  cfblk2 : Outport
  cfblk11 : Outport  Port=2
  cfblk12 : Outport  Port=3
  wires:
  cfblk7/1 -> cfblk5/1
  cfblk9/2(cfblk15) -> cfblk10/1(cfblk1)
  cfblk4/1 -> cfblk8/2(cfblk14)
  cfblk1/1 -> cfblk12/1
  cfblk6/1 -> cfblk5/2, cfblk9/6(cfblk14)
  cfblk9/3(cfblk16) -> cfblk11/1
  cfblk8/1(cfblk2) -> cfblk9/1(cfblk1)
  cfblk3/1 -> cfblk2/1
  cfblk8/2(cfblk15) -> cfblk3/1
  cfblk5/1 -> cfblk9/2(cfblk10), cfblk10/2(cfblk8), cfblk10/3(cfblk9)
  cfblk8/3(cfblk16) -> cfblk9/3(cfblk11)
  cfblk9/1(cfblk2) -> cfblk13/1
  cfblk13/1 -> cfblk8/1(cfblk1)
  cfblk10/1(cfblk2) -> cfblk14/1
  cfblk14/1 -> cfblk4/1
  cfblk10/2(cfblk10) -> cfblk15/1
  cfblk15/1 -> cfblk9/4(cfblk12)
  cfblk10/3(cfblk11) -> cfblk16/1
  cfblk16/1 -> cfblk9/5(cfblk13)

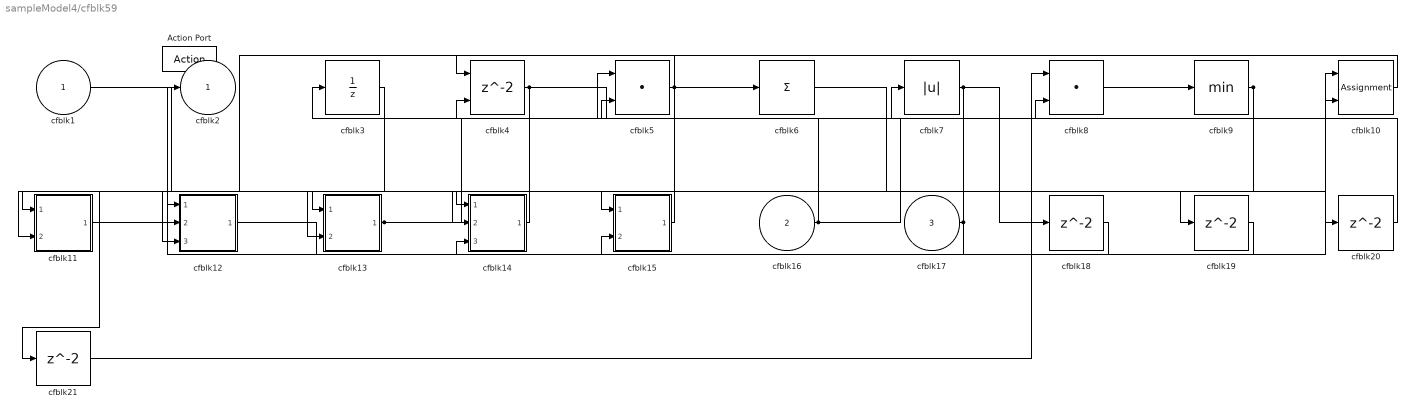
== system sampleModel4/cfblk59 ==
  cfblk1 : Inport
  cfblk16 : Inport  Port=2
  cfblk17 : Inport  Port=3
  Action Port : ActionPort  ActionPortLabel=if(u1 >= 0)
  cfblk10 : Assignment  DiagnosticForDimensions=Warning  IndexOptions=Index vector (dialog)  Indices=1  OutputSizes=1
  cfblk11 : Subsystem
  cfblk12 : Subsystem
  cfblk13 : Subsystem
  cfblk14 : Subsystem
  cfblk15 : Subsystem
  cfblk{18..21} (4 alike) : Delay
  cfblk3 : UnitDelay  SampleTime=-1  HasFrameUpgradeWarning=on
  cfblk4 : Delay  ShowEnablePort=on
      settings: InputPortMap=u0,e6
  cfblk5 : DotProduct  OutDataTypeStr=Inherit: Inherit via internal rule
  cfblk6 : Sum  Inputs=+
  cfblk7 : Abs  SaturateOnIntegerOverflow=off
  cfblk8 : DotProduct  OutDataTypeStr=Inherit: Inherit via internal rule
  cfblk9 : MinMax
  cfblk2 : Outport
  wires:
  cfblk16/1 -> cfblk3/1, cfblk8/2
  cfblk10/1 -> cfblk11/1(cfblk1)
  cfblk8/1 -> cfblk9/1
  cfblk12/1(cfblk2) -> cfblk10/1
  cfblk4/1 -> cfblk10/2, cfblk12/1(cfblk1)
  cfblk13/1(cfblk2) -> cfblk7/1, cfblk19/1
  cfblk3/1 -> cfblk11/2(cfblk10)
  cfblk15/1(cfblk2) -> cfblk14/1(cfblk1)
  cfblk5/1 -> cfblk14/2(cfblk11), cfblk4/1, cfblk6/1, cfblk12/3(cfblk14)
  cfblk17/1 -> cfblk5/2, cfblk12/2(cfblk13)
  cfblk7/1 -> cfblk4/2, cfblk18/1
  cfblk1/1 -> cfblk15/1(cfblk1)
  cfblk14/1(cfblk2) -> cfblk13/1(cfblk1)
  cfblk9/1 -> cfblk13/2(cfblk8), cfblk21/1
  cfblk11/1(cfblk2) -> cfblk2/1
  cfblk18/1 -> cfblk14/3(cfblk12)
  cfblk19/1 -> cfblk15/2(cfblk11)
  cfblk6/1 -> cfblk20/1
  cfblk20/1 -> cfblk5/1
  cfblk21/1 -> cfblk8/1

== system sampleModel4/cfblk60 ==
  cfblk1 : Inport
  cfblk8 : Inport  Port=2
  cfblk9 : Inport  Port=3
  Action Port : ActionPort  ActionPortLabel=else
  cfblk10 : Delay
  cfblk11 : Delay
  cfblk3 : DiscreteTransferFcn
  cfblk4 : Sum  Inputs=|++
  cfblk5 : Subsystem
  cfblk6 : Subsystem
  cfblk7 : Subsystem
  cfblk2 : Outport
  wires:
  cfblk1/1 -> cfblk7/1(cfblk1)
  cfblk9/1 -> cfblk5/1(cfblk1)
  cfblk8/1 -> cfblk7/2(cfblk11)
  cfblk5/1(cfblk2) -> cfblk2/1
  cfblk6/1(cfblk2) -> cfblk4/1
  cfblk3/1 -> cfblk6/2(cfblk8), cfblk5/4(cfblk8), cfblk10/1
  cfblk7/1(cfblk2) -> cfblk5/2(cfblk6)
  cfblk7/2(cfblk13) -> cfblk5/3(cfblk7)
  cfblk7/3(cfblk14) -> cfblk3/1
  cfblk7/4(cfblk15) -> cfblk4/2, cfblk5/5(cfblk9)
  cfblk10/1 -> cfblk7/3(cfblk12)
  cfblk4/1 -> cfblk11/1
  cfblk11/1 -> cfblk6/1(cfblk1)

== system sampleModel4/cfblk61 ==
  cfblk1 : Inport
  cfblk7 : Inport  Port=2
  Action Port : ActionPort  ActionPortLabel=if(u1 >= 0)
  cfblk3 : Rounding
  cfblk4 : Sqrt
  cfblk5 : MinMax  Function=max
  cfblk6 : Subsystem
  cfblk2 : Outport
  cfblk8 : Outport  Port=2
  wires:
  cfblk4/1 -> cfblk8/1
  cfblk5/1 -> cfblk4/1
  cfblk7/1 -> cfblk3/1
  cfblk1/1 -> cfblk6/1(cfblk1)
  cfblk3/1 -> cfblk5/1
  cfblk6/1(cfblk2) -> cfblk2/1

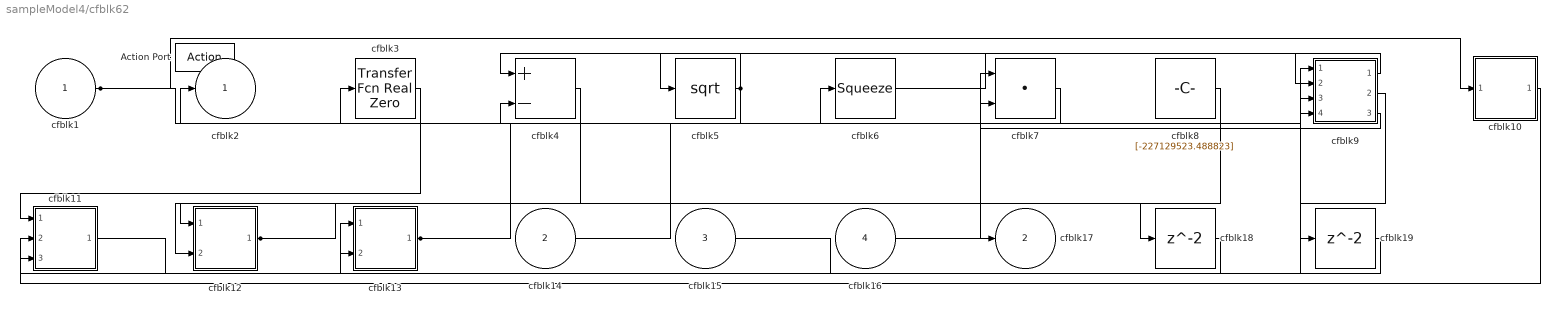
== system sampleModel4/cfblk62 ==
  cfblk1 : Inport
  cfblk14 : Inport  Port=2
  cfblk15 : Inport  Port=3
  cfblk16 : Inport  Port=4
  Action Port : ActionPort  ActionPortLabel=else
  cfblk10 : Subsystem
  cfblk11 : Subsystem
  cfblk12 : Subsystem
  cfblk13 : Subsystem
  cfblk18 : Delay
  cfblk19 : Delay
  cfblk3 : simulink/Discrete/Transfer Fcn Real Zero  ZeroZ=0.75  ICPrevInput=0.0  DoSatur=off
      settings: SourceProductBaseCode=SL
  cfblk4 : Sum  Inputs=+-
  cfblk5 : Sqrt
  cfblk6 : Squeeze
  cfblk7 : DotProduct  OutDataTypeStr=Inherit: Inherit via internal rule
  cfblk8 : Constant  Value=[-227129523.488823]  SampleTime=1
  cfblk9 : Subsystem
  cfblk2 : Outport
  cfblk17 : Outport  Port=2
  wires:
  cfblk8/1 -> cfblk12/1(cfblk1)
  cfblk15/1 -> cfblk9/1(cfblk1)
  cfblk1/1 -> cfblk10/1(cfblk1), cfblk3/1
  cfblk5/1 -> cfblk4/1, cfblk4/2
  cfblk3/1 -> cfblk11/1(cfblk1)
  cfblk13/1(cfblk2) -> cfblk6/1, cfblk9/4(cfblk15)
  cfblk6/1 -> cfblk9/2(cfblk13)
  cfblk7/1 -> cfblk2/1
  cfblk16/1 -> cfblk7/1
  cfblk4/1 -> cfblk12/2(cfblk9)
  cfblk11/1(cfblk2) -> cfblk13/1(cfblk1)
  cfblk10/1(cfblk2) -> cfblk11/2(cfblk6)
  cfblk14/1 -> cfblk9/3(cfblk14)
  cfblk12/1(cfblk2) -> cfblk17/1, cfblk18/1
  cfblk9/1(cfblk2) -> cfblk5/1
  cfblk9/3(cfblk17) -> cfblk7/2
  cfblk18/1 -> cfblk11/3(cfblk7)
  cfblk9/2(cfblk16) -> cfblk19/1
  cfblk19/1 -> cfblk13/2(cfblk11)

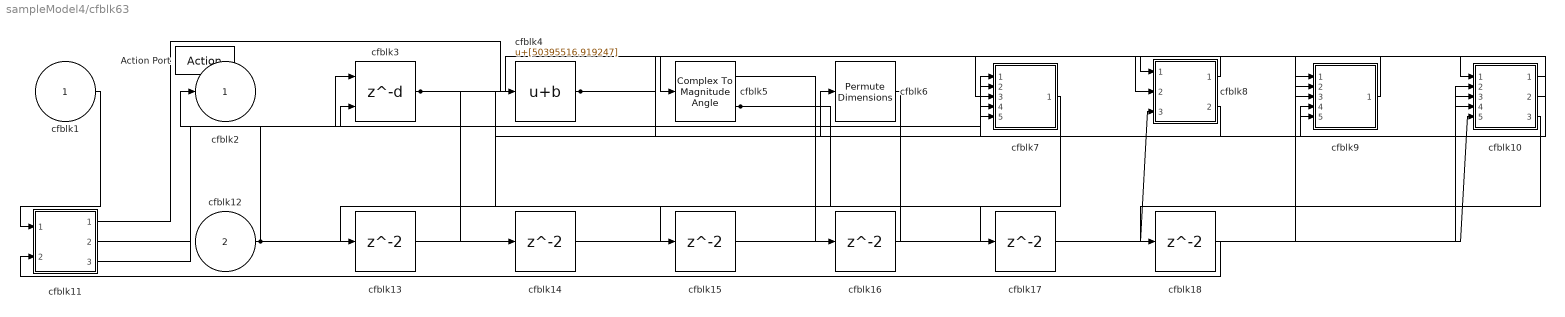
== system sampleModel4/cfblk63 ==
  cfblk1 : Inport
  cfblk12 : Inport  Port=2
  Action Port : ActionPort  ActionPortLabel=if(u1 >= 0)
  cfblk10 : Subsystem
  cfblk11 : Subsystem
  cfblk{13..18} (6 alike) : Delay
  cfblk3 : Delay  DelayLengthSource=Input port
      settings: InputPortMap=u0,p1
  cfblk4 : Bias  Bias=[50395516.919247]  SaturateOnIntegerOverflow=off
  cfblk5 : ComplexToMagnitudeAngle
  cfblk6 : PermuteDimensions
  cfblk7 : Subsystem
  cfblk8 : Subsystem
  cfblk9 : Subsystem
  cfblk2 : Outport
  wires:
  cfblk12/1 -> cfblk2/1, cfblk8/3(cfblk13), cfblk10/5(cfblk15)
  cfblk1/1 -> cfblk11/1(cfblk1)
  cfblk9/1(cfblk2) -> cfblk5/1
  cfblk10/1(cfblk2) -> cfblk6/1
  cfblk3/1 -> cfblk8/1(cfblk1), cfblk9/5(cfblk14), cfblk14/1, cfblk15/1
  cfblk6/1 -> cfblk3/2
  cfblk11/1(cfblk2) -> cfblk4/1
  cfblk5/2 -> cfblk7/1(cfblk1), cfblk17/1
  cfblk11/2(cfblk14) -> cfblk7/2(cfblk7)
  cfblk4/1 -> cfblk10/1(cfblk1), cfblk9/2(cfblk11), cfblk9/3(cfblk12), cfblk9/4(cfblk13)
  cfblk10/2(cfblk16) -> cfblk8/2(cfblk12)
  cfblk8/1(cfblk2) -> cfblk7/3(cfblk8)
  cfblk11/3(cfblk15) -> cfblk7/4(cfblk9)
  cfblk8/2(cfblk14) -> cfblk7/5(cfblk10)
  cfblk7/1(cfblk2) -> cfblk13/1
  cfblk13/1 -> cfblk10/2(cfblk12)
  cfblk14/1 -> cfblk10/3(cfblk13)
  cfblk15/1 -> cfblk10/4(cfblk14)
  cfblk5/1 -> cfblk16/1
  cfblk16/1 -> cfblk3/1
  cfblk17/1 -> cfblk9/1(cfblk1)
  cfblk10/3(cfblk17) -> cfblk18/1
  cfblk18/1 -> cfblk11/2(cfblk13)

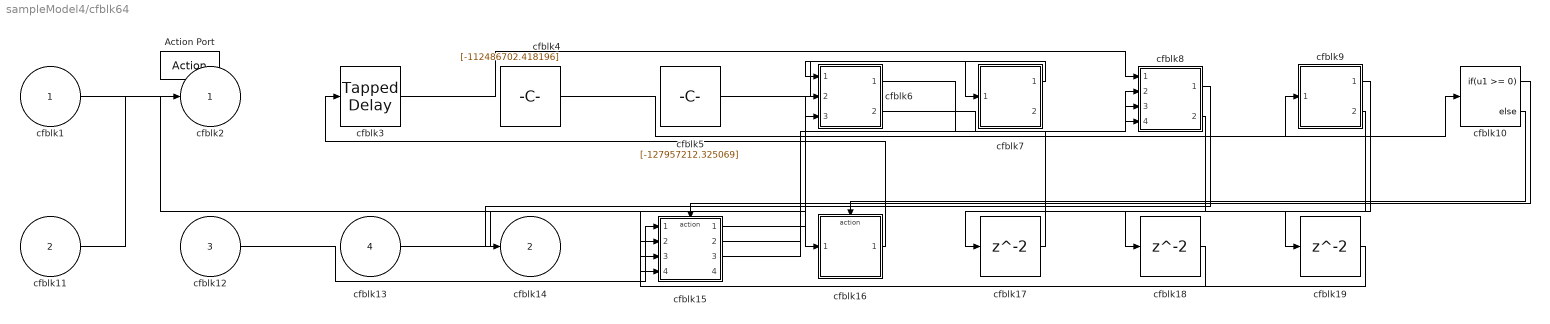
== system sampleModel4/cfblk64 ==
  cfblk1 : Inport
  cfblk11 : Inport  Port=2
  cfblk12 : Inport  Port=3
  cfblk13 : Inport  Port=4
  Action Port : ActionPort  ActionPortLabel=else
  cfblk10 : If  IfExpression=u1 >= 0  SampleTime=1
  cfblk15 : Subsystem  TreatAsAtomicUnit=on
  cfblk16 : Subsystem  TreatAsAtomicUnit=on
  cfblk17 : Delay
  cfblk18 : Delay
  cfblk19 : Delay
  cfblk3 : simulink/Discrete/Tapped Delay  vinit=0.0  samptime=-1  NumDelays=1  DelayOrder=Oldest  includeCurrent=off
  cfblk4 : Constant  Value=[-112486702.418196]  SampleTime=1
  cfblk5 : Constant  Value=[-127957212.325069]  SampleTime=1
  cfblk6 : Subsystem
  cfblk7 : Subsystem
  cfblk8 : Subsystem
  cfblk9 : Subsystem
  cfblk2 : Outport
  cfblk14 : Outport  Port=2
  wires:
  cfblk13/1 -> cfblk16/1(cfblk1)
  cfblk12/1 -> cfblk15/1(cfblk1)
  cfblk5/1 -> cfblk7/1(cfblk1)
  cfblk11/1 -> cfblk2/1
  cfblk3/1 -> cfblk8/1(cfblk1)
  cfblk4/1 -> cfblk10/1
  cfblk16/1(cfblk2) -> cfblk3/1
  cfblk7/1(cfblk2) -> cfblk6/1(cfblk1)
  cfblk6/1(cfblk2) -> cfblk8/2(cfblk14)
  cfblk6/2(cfblk9) -> cfblk8/3(cfblk15)
  cfblk15/1(cfblk2) -> cfblk6/2(cfblk7)
  cfblk8/1(cfblk2) -> cfblk14/1
  cfblk1/1 -> cfblk15/4(cfblk14)
  cfblk15/2(cfblk15) -> cfblk8/4(cfblk16)
  cfblk15/3(cfblk16) -> cfblk9/1(cfblk1)
  cfblk10/1 -> cfblk15/Action
  cfblk10/2 -> cfblk16/Action
  cfblk8/2(cfblk17) -> cfblk17/1
  cfblk17/1 -> cfblk6/3(cfblk8)
  cfblk9/1(cfblk2) -> cfblk18/1
  cfblk18/1 -> cfblk15/2(cfblk12)
  cfblk9/2(cfblk9) -> cfblk19/1
  cfblk19/1 -> cfblk15/3(cfblk13)

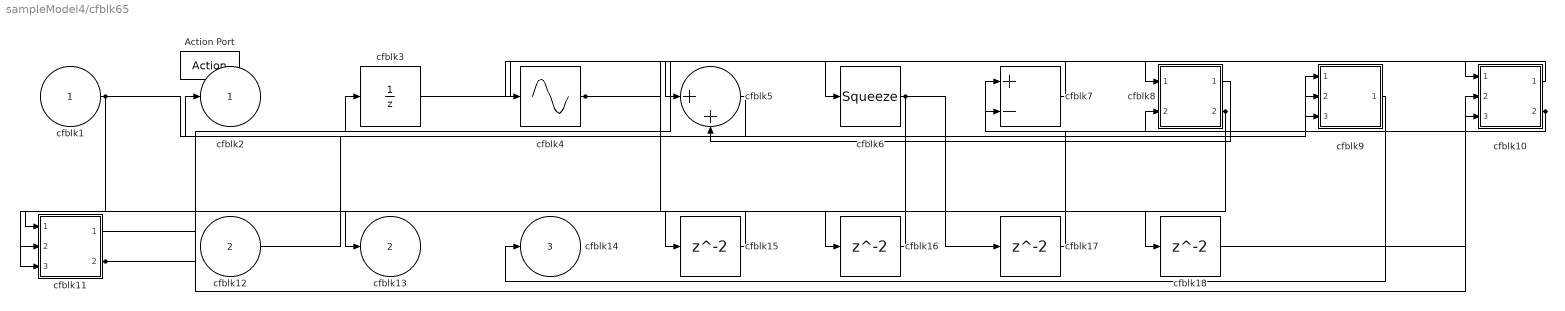
== system sampleModel4/cfblk65 ==
  cfblk1 : Inport
  cfblk12 : Inport  Port=2
  Action Port : ActionPort  ActionPortLabel=if(u1 >= 0)
  cfblk10 : Subsystem
  cfblk11 : Subsystem
  cfblk{15..18} (4 alike) : Delay
  cfblk3 : UnitDelay  SampleTime=-1  HasFrameUpgradeWarning=on
  cfblk4 : Sin  TimeSource=Use external signal  SampleTime=0
  cfblk5 : Sum  Inputs=|++
  cfblk6 : Squeeze
  cfblk7 : Sum  Inputs=+-
  cfblk8 : Subsystem
  cfblk9 : Subsystem
  cfblk2 : Outport
  cfblk13 : Outport  Port=2
  cfblk14 : Outport  Port=3
  wires:
  cfblk6/1 -> cfblk13/1, cfblk16/1, cfblk17/1
  cfblk11/1(cfblk2) -> cfblk10/1(cfblk1)
  cfblk5/1 -> cfblk2/1
  cfblk9/1(cfblk2) -> cfblk14/1
  cfblk11/2(cfblk9) -> cfblk10/2(cfblk6), cfblk3/1
  cfblk12/1 -> cfblk9/1(cfblk1)
  cfblk1/1 -> cfblk9/2(cfblk11), cfblk11/3(cfblk8)
  cfblk3/1 -> cfblk5/1
  cfblk7/1 -> cfblk4/1
  cfblk4/1 -> cfblk6/1, cfblk18/1
  cfblk10/1(cfblk2) -> cfblk8/1(cfblk1)
  cfblk8/1(cfblk2) -> cfblk5/2
  cfblk8/2(cfblk16) -> cfblk7/1, cfblk15/1
  cfblk10/2(cfblk8) -> cfblk9/3(cfblk12), cfblk8/2(cfblk15)
  cfblk15/1 -> cfblk11/1(cfblk1)
  cfblk16/1 -> cfblk11/2(cfblk7)
  cfblk17/1 -> cfblk7/2
  cfblk18/1 -> cfblk10/3(cfblk7)

== system sampleModel4/cfblk66 ==
  cfblk1 : Inport
  cfblk8 : Inport  Port=2
  cfblk9 : Inport  Port=3
  Action Port : ActionPort  ActionPortLabel=else
  cfblk10 : Delay
  cfblk11 : Delay
  cfblk3 : Delay
  cfblk4 : simulink/Math Operations/MinMax Running Resettable  Function=min  vinit=0.0
  cfblk5 : MinMax  Function=max
  cfblk6 : Constant  Value=[949359934.835099]  SampleTime=1
  cfblk7 : Subsystem
  cfblk2 : Outport
  wires:
  cfblk9/1 -> cfblk7/1(cfblk1), cfblk7/5(cfblk14)
  cfblk3/1 -> cfblk5/1
  cfblk4/1 -> cfblk2/1
  cfblk6/1 -> cfblk7/2(cfblk11)
  cfblk8/1 -> cfblk4/1
  cfblk1/1 -> cfblk4/2, cfblk7/4(cfblk13)
  cfblk5/1 -> cfblk10/1, cfblk11/1
  cfblk7/1(cfblk2) -> cfblk3/1
  cfblk10/1 -> cfblk7/3(cfblk12)
  cfblk11/1 -> cfblk7/6(cfblk15)

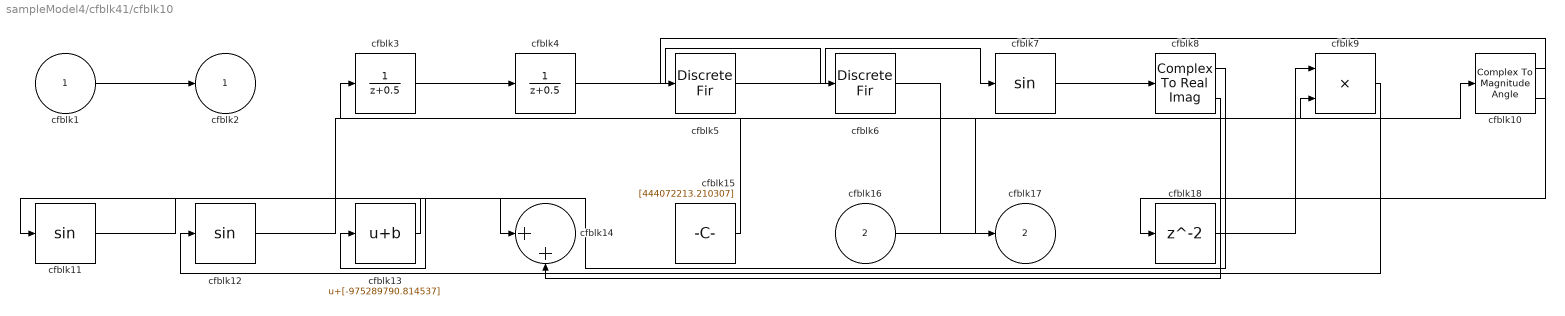
== system sampleModel4/cfblk41/cfblk10 ==
  cfblk1 : Inport
  cfblk16 : Inport  Port=2
  cfblk10 : ComplexToMagnitudeAngle
  cfblk11 : Trigonometry
  cfblk12 : Trigonometry
  cfblk13 : Bias  Bias=[-975289790.814537]  SaturateOnIntegerOverflow=off
  cfblk14 : Sum  Inputs=|++
  cfblk15 : Constant  Value=[444072213.210307]  SampleTime=1
  cfblk18 : Delay  SampleTime=1
  cfblk3 : DiscreteTransferFcn  SampleTime=1
  cfblk4 : DiscreteTransferFcn  SampleTime=1
  cfblk5 : DiscreteFir  SampleTime=1
  cfblk6 : DiscreteFir  SampleTime=1
  cfblk7 : Trigonometry
  cfblk8 : ComplexToRealImag
  cfblk9 : Product
  cfblk2 : Outport
  cfblk17 : Outport  Port=2
  wires:
  cfblk5/1 -> cfblk7/1
  cfblk15/1 -> cfblk3/1
  cfblk13/1 -> cfblk11/1
  cfblk4/1 -> cfblk6/1
  cfblk1/1 -> cfblk2/1
  cfblk7/1 -> cfblk8/1
  cfblk9/1 -> cfblk12/1
  cfblk6/1 -> cfblk17/1
  cfblk8/1 -> cfblk13/1
  cfblk11/1 -> cfblk14/1
  cfblk10/2 -> cfblk5/1
  cfblk16/1 -> cfblk9/2
  cfblk12/1 -> cfblk10/1
  cfblk3/1 -> cfblk4/1
  cfblk8/2 -> cfblk14/2
  cfblk10/1 -> cfblk18/1
  cfblk18/1 -> cfblk9/1

== system sampleModel4/cfblk41/cfblk11 ==
  cfblk1 : Inport
  cfblk10 : Inport  Port=2
  cfblk3 : Delay  SampleTime=1
  cfblk4 : DiscreteFir  SampleTime=1
  cfblk5 : Trigonometry
  cfblk6 : Sqrt
  cfblk7 : Sin  TimeSource=Use external signal  SampleTime=0
  cfblk8 : Constant  Value=[134879767.758352]  SampleTime=1
  cfblk9 : Constant  Value=[-148970890.124615]  SampleTime=1
  cfblk2 : Outport
  cfblk11 : Outport  Port=2
  wires:
  cfblk10/1 -> cfblk7/1
  cfblk8/1 -> cfblk6/1
  cfblk3/1 -> cfblk4/1
  cfblk7/1 -> cfblk5/1
  cfblk5/1 -> cfblk3/1
  cfblk6/1 -> cfblk2/1
  cfblk9/1 -> cfblk11/1

== system sampleModel4/cfblk42/cfblk7 ==
  cfblk1 : Inport
  cfblk9 : Inport  Port=2
  cfblk10 : Inport  Port=3
  cfblk3 : Delay  DelayLengthSource=Input port  SampleTime=1
      settings: InputPortMap=u0,p1
  cfblk4 : simulink/Discrete/Transfer Fcn First Order  PoleZ=0.95  ICPrevOutput=0.0  DoSatur=off
  cfblk5 : Sin  TimeSource=Use external signal  SampleTime=0
  cfblk6 : Product  Inputs=*
  cfblk7 : Product  Inputs=**
  cfblk8 : Constant  Value=[496883942.061240]  SampleTime=1
  cfblk2 : Outport
  wires:
  cfblk1/1 -> cfblk4/1
  cfblk8/1 -> cfblk6/1
  cfblk4/1 -> cfblk2/1
  cfblk5/1 -> cfblk3/1
  cfblk6/1 -> cfblk3/2
  cfblk9/1 -> cfblk5/1
  cfblk3/1 -> cfblk7/1
  cfblk10/1 -> cfblk7/2

== system sampleModel4/cfblk42/cfblk8 ==
  cfblk1 : Inport
  cfblk11 : Inport  Port=2
  cfblk10 : Product  Inputs=*
  cfblk3 : Delay  ShowEnablePort=on  SampleTime=1
      settings: InputPortMap=u0,e6
  cfblk4 : UnitDelay  HasFrameUpgradeWarning=on
  cfblk5 : UnitDelay  HasFrameUpgradeWarning=on
  cfblk6 : Squeeze
  cfblk7 : ComplexToRealImag
  cfblk8 : MinMax
  cfblk9 : Sum  Inputs=+
  cfblk2 : Outport
  cfblk12 : Outport  Port=2
  cfblk13 : Outport  Port=3
  cfblk14 : Outport  Port=4
  wires:
  cfblk3/1 -> cfblk9/1
  cfblk9/1 -> cfblk14/1
  cfblk6/1 -> cfblk12/1
  cfblk10/1 -> cfblk13/1
  cfblk11/1 -> cfblk2/1
  cfblk4/1 -> cfblk7/1
  cfblk8/1 -> cfblk10/1
  cfblk5/1 -> cfblk6/1, cfblk4/1, cfblk3/2
  cfblk7/1 -> cfblk3/1
  cfblk7/2 -> cfblk8/1
  cfblk1/1 -> cfblk5/1
